simulink model "SmartACController"  (R2025a)
settings: Solver=FixedStepDiscrete  StartTime=0.0  StopTime=300  FixedStep=0.01  RelTol=1e-3
settings Model: Creator=wangtianqi  LastModifiedBy=wangtianqi

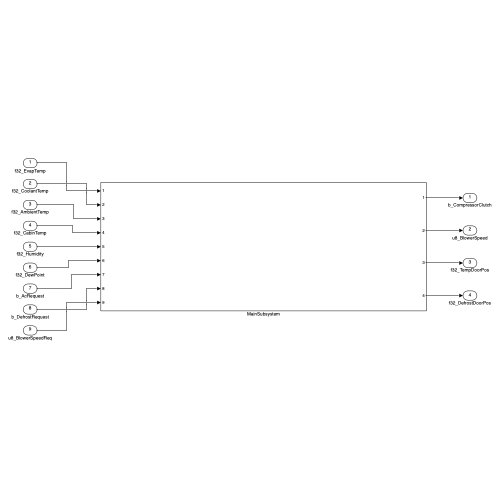
[thumbnail: Simulink's stored preview of the top-level diagram]
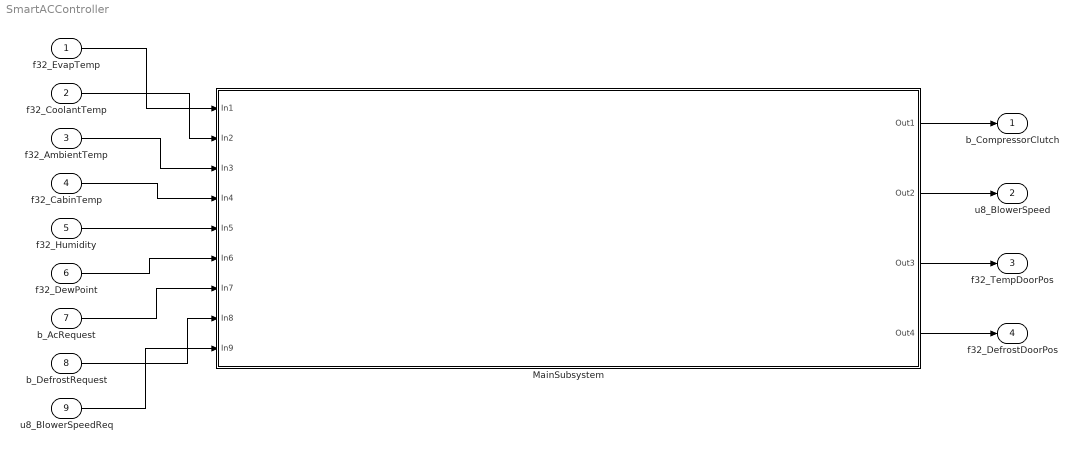
== system SmartACController ==
  f32_EvapTemp : Inport  OutDataTypeStr=single
  f32_CoolantTemp : Inport  Port=2  OutDataTypeStr=single
  f32_AmbientTemp : Inport  Port=3  OutDataTypeStr=single
  f32_CabinTemp : Inport  Port=4  OutDataTypeStr=single
  f32_Humidity : Inport  Port=5  OutDataTypeStr=single
  f32_DewPoint : Inport  Port=6  OutDataTypeStr=single
  b_AcRequest : Inport  Port=7  OutDataTypeStr=single
  b_DefrostRequest : Inport  Port=8  OutDataTypeStr=single
  u8_BlowerSpeedReq : Inport  Port=9  OutDataTypeStr=single
  MainSubsystem : Subsystem
  b_CompressorClutch : Outport  OutDataTypeStr=boolean
  u8_BlowerSpeed : Outport  Port=2  OutDataTypeStr=uint8
  f32_TempDoorPos : Outport  Port=3  OutDataTypeStr=single
  f32_DefrostDoorPos : Outport  Port=4  OutDataTypeStr=single
  wires:
  MainSubsystem/4(Out4) -> f32_DefrostDoorPos/1
  MainSubsystem/3(Out3) -> f32_TempDoorPos/1
  u8_BlowerSpeedReq/1 -> MainSubsystem/9(In9)
  b_AcRequest/1 -> MainSubsystem/7(In7)
  MainSubsystem/2(Out2) -> u8_BlowerSpeed/1
  b_DefrostRequest/1 -> MainSubsystem/8(In8)
  f32_DewPoint/1 -> MainSubsystem/6(In6)
  f32_Humidity/1 -> MainSubsystem/5(In5)
  f32_CabinTemp/1 -> MainSubsystem/4(In4)
  f32_AmbientTemp/1 -> MainSubsystem/3(In3)
  f32_CoolantTemp/1 -> MainSubsystem/2(In2)
  MainSubsystem/1(Out1) -> b_CompressorClutch/1
  f32_EvapTemp/1 -> MainSubsystem/1(In1)

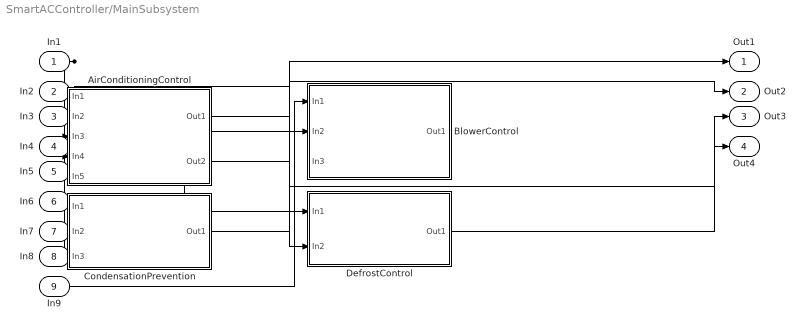
== system SmartACController/MainSubsystem ==
  In1 : Inport
  In2 : Inport  Port=2
  In3 : Inport  Port=3
  In4 : Inport  Port=4
  In5 : Inport  Port=5
  In6 : Inport  Port=6
  In7 : Inport  Port=7
  In8 : Inport  Port=8
  In9 : Inport  Port=9
  AirConditioningControl : Subsystem
  BlowerControl : Subsystem
  CondensationPrevention : Subsystem
  DefrostControl : Subsystem
  Out1 : Outport
  Out2 : Outport  Port=2
  Out3 : Outport  Port=3
  Out4 : Outport  Port=4
  wires:
  In1/1 -> AirConditioningControl/1(In1), CondensationPrevention/1(In1)
  In2/1 -> AirConditioningControl/2(In2), DefrostControl/2(In2)
  In4/1 -> AirConditioningControl/3(In3)
  In7/1 -> AirConditioningControl/4(In4), BlowerControl/2(In2)
  In5/1 -> AirConditioningControl/5(In5), CondensationPrevention/2(In2)
  In6/1 -> CondensationPrevention/3(In3)
  In9/1 -> BlowerControl/1(In1)
  In8/1 -> DefrostControl/1(In1)
  AirConditioningControl/1(Out1) -> Out1/1
  AirConditioningControl/2(Out2) -> Out2/1
  CondensationPrevention/1(Out1) -> Out3/1
  DefrostControl/1(Out1) -> Out4/1

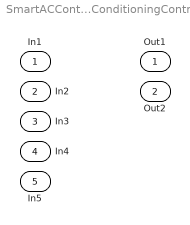
== system SmartACController/MainSubsystem/AirConditioningControl ==
  In1 : Inport
  In2 : Inport  Port=2
  In3 : Inport  Port=3
  In4 : Inport  Port=4
  In5 : Inport  Port=5
  Out1 : Outport
  Out2 : Outport  Port=2

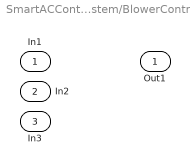
== system SmartACController/MainSubsystem/BlowerControl ==
  In1 : Inport
  In2 : Inport  Port=2
  In3 : Inport  Port=3
  Out1 : Outport

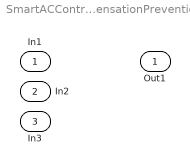
== system SmartACController/MainSubsystem/CondensationPrevention ==
  In1 : Inport
  In2 : Inport  Port=2
  In3 : Inport  Port=3
  Out1 : Outport

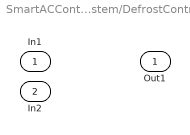
== system SmartACController/MainSubsystem/DefrostControl ==
  In1 : Inport
  In2 : Inport  Port=2
  Out1 : Outport
